simulink model "LUPA2body"  (R2024b)
settings: Solver=ode4  StartTime=0  StopTime=60  FixedStep=0.01  MaxStep=0.01  RelTol=1e-3
values from neighbouring files (symbols this model uses):
  Ki = -3816    [wecSimInputFile.m]
  Kp = 1034    [wecSimInputFile.m]
undefined symbols (not defined in the file or in its folder): body, constraint, geometry, hydroData, pto
libraries: WECSim_Lib_Body_Elements x2, WECSim_Lib_Constraints x1, WECSim_Lib_Frames x1, WECSim_Lib_PTOs x1
settings Model: Creator=Bosma  LastModifiedBy=bosmab
settings SolverCC: ConcurrentTasks=on  ZeroCrossControl=DisableAll  PositivePriorityOrder=on  AutoInsertRateTranBlk=on
settings DataIOCC: ReturnWorkspaceOutputs=off
settings OptimizationCC: BlockReduction=off  OptimizeBlockIOStorage=off  SimCompilerOptimization=on
settings DebuggingCC: TasksWithSamePriorityMsg=none
settings HardwareCC: ProdBitPerLong=64  ProdLongLongMode=on  ProdHWDeviceType=Intel->x86-64 (Linux 64)
settings SFSimCC: SimTargetLang=C++
settings RTWCC: Description=Speedgoat Real-Time Target Machine  SystemTargetFile=speedgoat.tlc  TemplateMakefile=slrealtime_default_tmf  Toolchain=Simulink Real-Time Toolchain  BuildConfiguration=Faster Runs  CodeExecutionProfiling=on  TargetLang=C++  GPUComputeCapability=3.5
settings SimulinkRealTimeTargetCC: InstructionSetFMA=off  LogToMDFFile=off

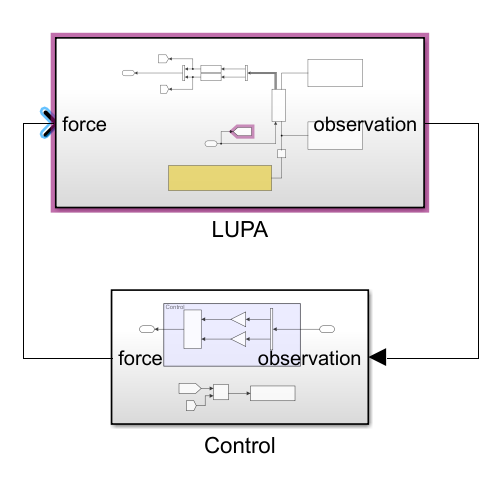
[thumbnail: Simulink's stored preview of the top-level diagram]
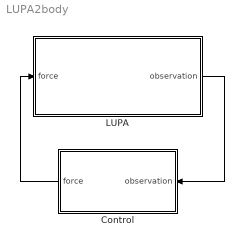
== system LUPA2body ==
  Control : Subsystem
  LUPA : Subsystem
  wires:
  LUPA/1(observation) -> Control/1(observation)
  Control/1(force) -> LUPA/1(force)

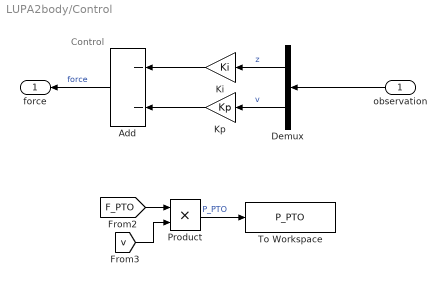
== system LUPA2body/Control ==
  note: Control
  observation : Inport
  Add : Sum  Inputs=--
  Demux : Demux  Outputs=2
  Ki : Gain  Gain=Ki
  Kp : Gain  Gain=Kp
  Product : Product
  To Workspace : ToWorkspace  VariableName=P_PTO  SaveFormat=Timeseries  SampleTime=-1
  force : Outport
  wires:
  [F_PTO] -> Product/1
  Product/1 -> To Workspace/1  "P_PTO"
  observation/1 -> Demux/1
  [v] -> Product/2
  Demux/1 -> Ki/1  "z"
  Demux/2 -> Kp/1  "v"
  Ki/1 -> Add/1
  Kp/1 -> Add/2
  Add/1 -> force/1  "force"

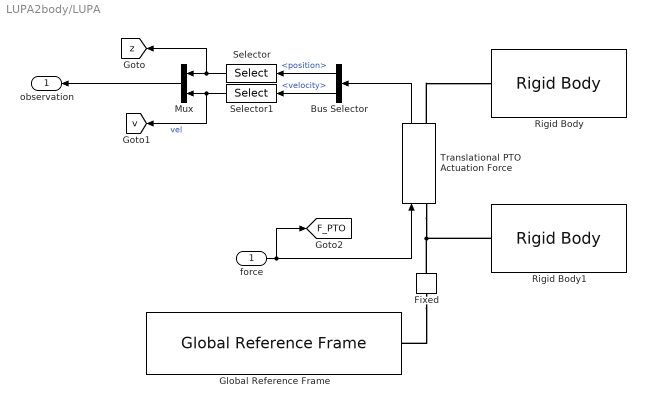
== system LUPA2body/LUPA ==
  force : Inport
  Bus Selector : BusSelector  OutputSignals=position,velocity
  Fixed : WECSim_Lib_Constraints/Fixed  constraint=constraint(1)  loc="0  0  0"  displacement=0 0 0  y=0 1 0  z=0 0 1  upperLimitSpecify=off  upperLimitBound=0  upperLimitTransitionRegionWidth=0  upperLimitStiffness=0  upperLimitDamping=0  lowerLimitSpecify=off  lowerLimitBound=0  lowerLimitTransitionRegionWidth=0  lowerLimitStiffness=0  lowerLimitDamping=0
      settings: AttributesFormatString=%<constraint>
  Global Reference Frame : WECSim_Lib_Frames/Global Reference Frame  waves=waves  simu=simu  InputMethod=Input File  InputFile=wecSimInputFile.m  mode=normal  explorer=off  solver=ode4  startTime=""  rampTime=100  endTime=400  dt=0.1  cicEndTime=60  stateSpace=0  WaveClass=regular  height=2.5  period=8  elevationFile=NOT DEFINED  spectrumFile=NOT DEFINED  direction=0  spread=1  spectrumType=NOT DEFINED  phaseSeed=0  option=EqualEnergy
  Mux : Mux  Inputs=2
  Rigid Body : WECSim_Lib_Body_Elements/Rigid Body  body=body(1)  h5File=hydroData/*.h5  geometryFile=geometry/*.stl  mass=0  inertia=0 0 0  inertiaProducts=0 0 0  nonHydro=0  nonlinearHydro=0  centerGravity=0 0 0  centerBuoyancy=0 0 0  dof=6  volume=0  QTFs=0  displacement=0 0 0  axis=0 1 0  angle=0  option=0  cd=0 0 0  ca=0 0 0  area=0 0 0  VME=0  rgME=0 0 0  z=0 0 1
  Rigid Body1 : WECSim_Lib_Body_Elements/Rigid Body  body=body(2)  h5File=hydroData/*.h5  geometryFile=geometry/*.stl  mass=0  inertia=0 0 0  inertiaProducts=0 0 0  nonHydro=0  nonlinearHydro=0  centerGravity=0 0 0  centerBuoyancy=0 0 0  dof=6  volume=0  QTFs=0  displacement=0 0 0  axis=0 1 0  angle=0  option=0  cd=0 0 0  ca=0 0 0  area=0 0 0  VME=0  rgME=0 0 0  z=0 0 1
  Selector : Selector  InputPortWidth=6  IndexOptions=Index vector (dialog)  Indices=[3]  OutputSizes=1
  Selector1 : Selector  InputPortWidth=6  IndexOptions=Index vector (dialog)  Indices=[3]  OutputSizes=1
  Translational PTO Actuation Force : WECSim_Lib_PTOs/Translational PTO Actuation Force  pto=pto(1)  loc="0  0  0"  stiffness=0  damping=0  equilibriumPosition=0  pretension=0  displacement=0 0 0  y=0 1 0  z=0 0 1  upperLimitSpecify=off  upperLimitBound=0  upperLimitTransitionRegionWidth=0  upperLimitStiffness=0  upperLimitDamping=0  lowerLimitSpecify=off  lowerLimitBound=0  lowerLimitTransitionRegionWidth=0  lowerLimitStiffness=0  lowerLimitDamping=0
      settings: AttributesFormatString=%<pto>
  observation : Outport
  tag scope: F_PTO=global, v=global, z=global
  wires:
  Selector/1 -> [z], Mux/1
  Selector1/1 -> [v], Mux/2  "vel"
  Bus Selector/2 -> Selector1/1  "<velocity>"
  Bus Selector/1 -> Selector/1  "<position>"
  Translational PTO Actuation Force/1 -> Bus Selector/1
  force/1 -> [F_PTO], Translational PTO Actuation Force/1
  Mux/1 -> observation/1
  connections:
  Fixed/LConn1 -- Global Reference Frame/RConn1
  Translational PTO Actuation Force/RConn1 -- Rigid Body/RConn1
  Rigid Body1/RConn1 -- Fixed/RConn1 -- Translational PTO Actuation Force/LConn1
